simulink model "QuadPID"  (Simulink 9.3)
settings: Solver=ode45  StartTime=0.0  StopTime=500  MaxStep=0.01  RelTol=1e-3  EnableMultiTasking=on
values from neighbouring files (symbols this model uses):
  Fd = 0    [Low_Fidelity_Model.m]
  g = 9.81    [Low_Fidelity_Model.m]    (also in make_graphs.m)
  h0 = hdes0    (= 0.7)    [Low_Fidelity_Model.m]
  hdes0 = 0.7    [Low_Fidelity_Model.m]
  hdesf = 1.25    [Low_Fidelity_Model.m]
  hdot0 = 0    [Low_Fidelity_Model.m]
  Kd = input('Enter the derivative gain, Kd: ')    [Low_Fidelity_Model.m]
  Ki = 0    [Low_Fidelity_Model.m]
  Kp = input('Enter the proportional gain, Kp: ')    [Low_Fidelity_Model.m]
  kT = input('Enter the estimated thrust coefficient, N, kT: ')    [Low_Fidelity_Model.m]
  kThat = kT    [Low_Fidelity_Model.m]
  m = 65e-3    (= 0.065)    [Low_Fidelity_Model.m]
  mhat = m    (= 0.065)    [Low_Fidelity_Model.m]
  tstep = 1    [Low_Fidelity_Model.m]
  umax = 500    [Low_Fidelity_Model.m]
  umin = 0    [Low_Fidelity_Model.m]
settings Model: Creator=pjseiler  LastModifiedBy=pjseiler
settings DataIOCC: LimitDataPoints=on
settings OptimizationCC: ExpressionDepthLimit=2147483647
settings DebuggingCC: SolverPrmCheckMsg=warning  StateNameClashWarn=warning  SFExecutionAtInitializationDiag=warning
settings GRTTargetCC: GeneratePreprocessorConditionals=Disable all

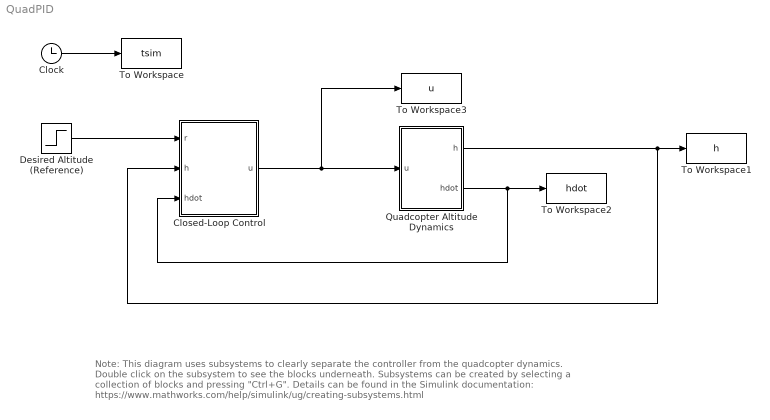
== system QuadPID ==
  note: Note: This diagram uses subsystems to clearly separate the controller from the quadcopter dynamics.
      | Double click on the subsystem to see the blocks underneath. Subsystems can be created by selecting
      | a collection of blocks and pressing "Ctrl+G". Details can be found in the Simulink documentation:
      | https://www.mathworks.com/help/simulink/ug/creating-subsystems.html
  Clock : Clock
  Closed-Loop Control : Subsystem
  Desired Altitude (Reference) : Step  Time=tstep  Before=hdes0  After=hdesf  SampleTime=0
  Quadcopter Altitude Dynamics : Subsystem
  To Workspace : ToWorkspace  VariableName=tsim  SampleTime=-1
  To Workspace1 : ToWorkspace  VariableName=h  SampleTime=-1
  To Workspace2 : ToWorkspace  VariableName=hdot  SampleTime=-1
  To Workspace3 : ToWorkspace  VariableName=u  SampleTime=-1
  wires:
  Clock/1 -> To Workspace/1
  Desired Altitude (Reference)/1 -> Closed-Loop Control/1(r)
  Closed-Loop Control/1(u) -> To Workspace3/1, Quadcopter Altitude Dynamics/1(u)
  Quadcopter Altitude Dynamics/1(h) -> Closed-Loop Control/2(h), To Workspace1/1
  Quadcopter Altitude Dynamics/2(hdot) -> Closed-Loop Control/3(hdot), To Workspace2/1

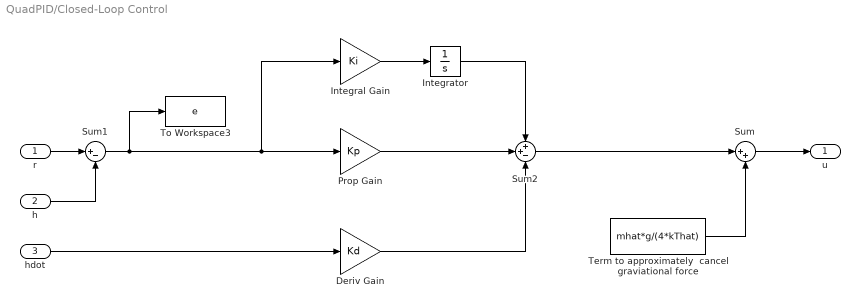
== system QuadPID/Closed-Loop Control ==
  r : Inport
  h : Inport  Port=2
  hdot : Inport  Port=3
  Deriv Gain : Gain  Gain=Kd
  Integral Gain : Gain  Gain=Ki
  Integrator : Integrator
  Prop Gain : Gain  Gain=Kp
  Sum : Sum  Inputs=|++
  Sum1 : Sum  Inputs=|+-
  Sum2 : Sum  Inputs=++-
  Term to approximately  cancel graviational force : Constant  Value=mhat*g/(4*kThat)
  To Workspace3 : ToWorkspace  VariableName=e  SampleTime=-1
  u : Outport
  wires:
  Sum/1 -> u/1
  Term to approximately  cancel graviational force/1 -> Sum/2
  r/1 -> Sum1/1
  Sum1/1 -> Integral Gain/1, Prop Gain/1, To Workspace3/1
  h/1 -> Sum1/2
  Integral Gain/1 -> Integrator/1
  Prop Gain/1 -> Sum2/2
  Sum2/1 -> Sum/1
  Integrator/1 -> Sum2/1
  hdot/1 -> Deriv Gain/1
  Deriv Gain/1 -> Sum2/3

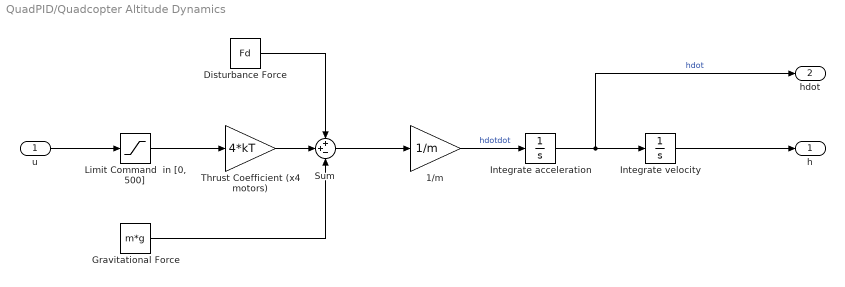
== system QuadPID/Quadcopter Altitude Dynamics ==
  u : Inport
  1/m : Gain  Gain=1/m
  Disturbance Force : Constant  Value=Fd
  Gravitational Force : Constant  Value=m*g
  Integrate acceleration : Integrator  InitialCondition=hdot0
  Integrate velocity : Integrator  InitialCondition=h0
  "Limit Command  in [0, 500]" : Saturate  UpperLimit=umax  LowerLimit=umin
  Sum : Sum  Inputs=++-
  Thrust Coefficient (x4 motors) : Gain  Gain=4*kT
  h : Outport
  hdot : Outport  Port=2
  wires:
  Integrate acceleration/1 -> hdot/1, Integrate velocity/1  "hdot"
  Sum/1 -> 1/m/1
  u/1 -> "Limit Command  in [0, 500]"/1
  "Limit Command  in [0, 500]"/1 -> Thrust Coefficient (x4 motors)/1
  1/m/1 -> Integrate acceleration/1  "hdotdot"
  Integrate velocity/1 -> h/1
  Gravitational Force/1 -> Sum/3
  Disturbance Force/1 -> Sum/1
  Thrust Coefficient (x4 motors)/1 -> Sum/2
